simulink model "practica"  (Simulink 4.00)
settings: Solver=ode45  StartTime=0.0  StopTime=100.0  FixedStep=.1  MaxStep=.1*ts  RelTol=1e-4
undefined symbols (not defined in the file): ts
settings Model: LimitDataPoints=off  ExtModeTrigMode=oneshot  ExtModeArmWhenConnect=off  BlockReductionOpt=off

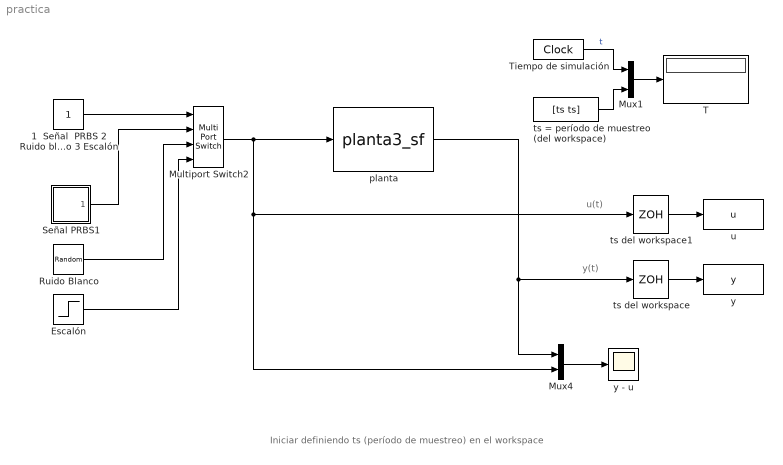
== system practica ==
  note: y(t)
  note: u(t)
  note: Iniciar definiendo ts (período de muestreo) en el workspace
  1  Señal  PRBS 2 Ruido blanco 3 Escalón : Constant  Value=1
  Escalón : Step  Time=0  Before=0  After=1  SampleTime=0
  Multiport Switch2 : MultiPortSwitch  Inputs=3
  Mux1 : Mux  Inputs=2
  Mux4 : Mux  Inputs=2
  Ruido Blanco : RandomNumber  Mean=0  Variance=1  Seed=0  SampleTime=0
  Señal PRBS1 : Subsystem
      settings: RTWFcnNameOpts=Auto  RTWFileNameOpts=Auto
  T : Display
      settings: Format=short
  Tiempo de simulación : DigitalClock  SampleTime=.1
  planta : S-Function  FunctionName=planta3_sf  PortCounts=[]  SFunctionModules=''
  ts = período de muestreo (del workspace) : FromWorkspace  VariableName=[ts ts]  SampleTime=0  OutputAfterFinalValue=Extrapolation
  ts del workspace : ZeroOrderHold  SampleTime=ts
  ts del workspace1 : ZeroOrderHold  SampleTime=ts
  u : ToWorkspace  VariableName=u  SampleTime=ts  SaveFormat=Array
  y : ToWorkspace  VariableName=y  SampleTime=ts  SaveFormat=Array
  y - u : Scope
      settings: TimeRange=auto  YMin=-5  YMax=5  SaveToWorkspace=off  MaxDataPoints=5000
  wires:
  1  Señal  PRBS 2 Ruido blanco 3 Escalón/1 -> Multiport Switch2/1
  Ruido Blanco/1 -> Multiport Switch2/3
  Mux4/1 -> y - u/1
  planta/1 -> ts del workspace/1, Mux4/1
  Multiport Switch2/1 -> planta/1, Mux4/2, ts del workspace1/1
  Escalón/1 -> Multiport Switch2/4
  Señal PRBS1/1(u ( t )) -> Multiport Switch2/2
  ts del workspace/1 -> y/1
  ts = período de muestreo (del workspace)/1 -> Mux1/2
  Tiempo de simulación/1 -> Mux1/1  "t"
  Mux1/1 -> T/1
  ts del workspace1/1 -> u/1

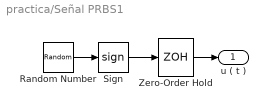
== system practica/Señal PRBS1 ==
  Random Number : RandomNumber  Mean=0  Variance=1  Seed=0  SampleTime=0
  Sign : Signum
  Zero-Order Hold : ZeroOrderHold  SampleTime=ts
  u ( t ) : Outport  Port=1
  wires:
  Zero-Order Hold/1 -> u ( t )/1
  Sign/1 -> Zero-Order Hold/1
  Random Number/1 -> Sign/1
